simulink model "gm_uz_mpc_6ph"  (R2021a)
settings: Solver=FixedStepDiscrete  StartTime=0.0  StopTime=200*t_ADC  RelTol=1e-3
undefined symbols (not defined in the file or in its folder): IB, id_ref, iq_ref, ix_ref, iy_ref, lambda_d, lambda_q, lambda_u, lambda_x, lambda_y, Ld_over_LB, Lq_over_LB, n_rpm, omegaB, p, psi_pm_over_psiB, Rs_over_ZB, t_ADC, t_clock, Ts_times_ZB_over_Ld, Ts_times_ZB_over_Lq, Ts_times_ZB_over_Lx, Ts_times_ZB_over_Ly, v_dc, VB
libraries: nesl_utility x32, fl_lib x29, simulink x21, ee_lib x12, hdlsllib x2, spsAlphaBetaZerotodq0Lib x1
(part 2 of 4)

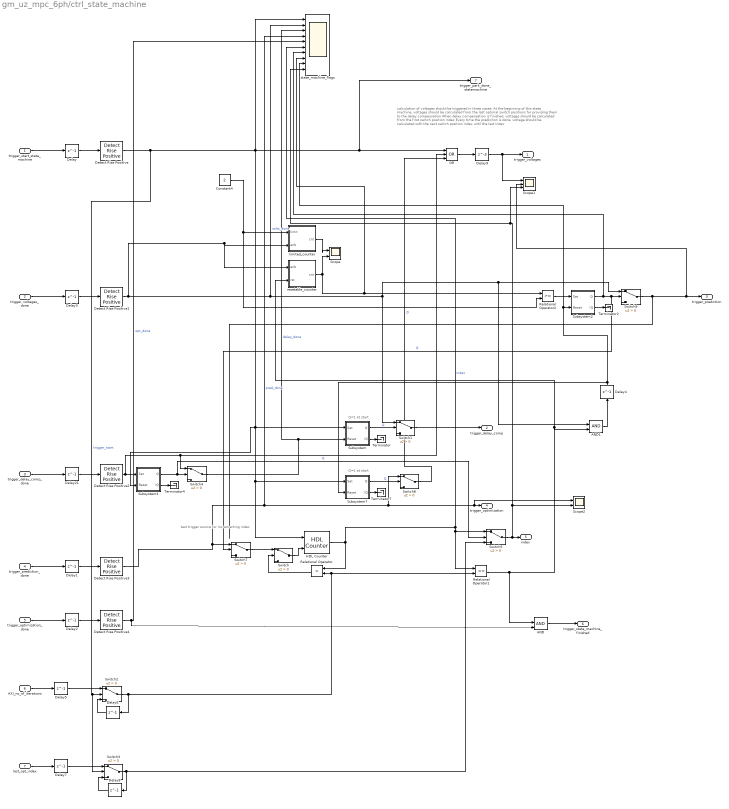
== system gm_uz_mpc_6ph/ctrl_state_machine ==
  note: Q=1 at start
  note: Q=1 at start
  note: calculation of voltages should be triggered in three cases:
      |
      | At the beginning of this state machine, voltages should be calculated from the last optimal switch positions for providing them to the delay compensation
      | When delay compensation is finished, voltages should be calculated from the first switch position index
      | Every time the prediciton is done, voltage should be calculated with the next switch position index until the last index
  note: test trigger source for incrementing index
  trigger_start_state_machine : Inport
  trigger_voltages_done : Inport  Port=2
  trigger_delay_comp_done : Inport  Port=3
  trigger_prediction_done : Inport  Port=4
  trigger_optimization_done : Inport  Port=5
  AXI_no_of_iterations : Inport  Port=6  OutDataTypeStr=uint32
  last_opt_index : Inport  Port=7  OutDataTypeStr=uint32
  AND : Logic  IconShape=distinctive  AllPortsSameDT=off  OutDataTypeStr=boolean
  AND1 : Logic  IconShape=distinctive  AllPortsSameDT=off  OutDataTypeStr=boolean
  Constant4 : Constant  Value=2  OutDataTypeStr=uint8  SampleTime=-1
  Delay{,1..8,21} (10 alike) : Delay  DelayLength=1
  Delay9 : Delay  DelayLength=3
  Detect Rise Positive{,1..4} (5 alike) : simulink/Logic and Bit Operations/Detect Rise Positive  vinit=0  OutDataTypeStr=boolean
  HDL Counter : hdlsllib/Sources/HDL Counter  CountType=Free running  CountInit=1  CountStep=1  CountMax=25  CountFromType=Initial value  CountFrom=1  CountResetPort=on  CountLoadPort=off  CountEnbPort=on  CountDirPort=off  CountHitOutputPort=off  CountDataType=Unsigned  CountWordLen=32  CountFracLen=0  CountSampTime=1
  OR : Logic  Operator=OR  Inputs=3  IconShape=distinctive  AllPortsSameDT=off  OutDataTypeStr=boolean
  Relational Operator : RelationalOperator  Operator=<  OutDataTypeStr=boolean  RndMeth=Simplest
  Relational Operator1 : RelationalOperator  Operator===  OutDataTypeStr=boolean  RndMeth=Simplest
  Relational Operator2 : RelationalOperator  OutDataTypeStr=boolean  RndMeth=Simplest
  Scope : Scope  NumInputPorts=2
  Scope1 : Scope  NumInputPorts=3
  Scope2 : Scope  NumInputPorts=2
  Subsystem : Subsystem
  Subsystem2 : Subsystem
  Subsystem4 : Subsystem
  Subsystem7 : Subsystem
  Switch{,1..5,7..9} (9 alike) : Switch  Criteria=u2 > Threshold
  Terminator{,2,4,7} (4 alike) : Terminator
  limited_counter : Subsystem
  resetable_counter : Subsystem
  state_machine_flags : Scope  NumInputPorts=10
  trigger_voltages : Outport  VectorParamsAs1DForOutWhenUnconnected=off
  trigger_delay_comp : Outport  Port=2  VectorParamsAs1DForOutWhenUnconnected=off
  trigger_prediction : Outport  Port=3  VectorParamsAs1DForOutWhenUnconnected=off
  trigger_optimization : Outport  Port=4  VectorParamsAs1DForOutWhenUnconnected=off
  index : Outport  Port=5  VectorParamsAs1DForOutWhenUnconnected=off
  trigger_state_machine_finished : Outport  Port=6  VectorParamsAs1DForOutWhenUnconnected=off
  trigger_park_done_statemachine : Outport  Port=7  VectorParamsAs1DForOutWhenUnconnected=off
  wires:
  Delay9/1 -> trigger_voltages/1, Scope1/1
  OR/1 -> Delay9/1
  Switch5/1 -> index/1, Scope2/2, state_machine_flags/10, Scope1/3
  Delay8/1 -> Switch3/3
  Delay7/1 -> Switch3/1
  Switch3/1 -> Delay8/1, Switch5/3
  last_opt_index/1 -> Delay7/1
  Delay6/1 -> Switch2/3
  Delay5/1 -> Switch2/1
  AXI_no_of_iterations/1 -> Delay5/1
  Subsystem7/1(Q) -> Switch8/2  "Q"
  Subsystem7/2(!Q) -> Terminator7/1
  Switch8/1 -> OR/3  "Q"
  Delay4/1 -> Subsystem7/2(Reset), Subsystem2/2(Reset), state_machine_flags/9
  AND1/1 -> Delay4/1
  AND/1 -> trigger_state_machine_finished/1
  Switch9/1 -> trigger_prediction/1, Scope1/2
  Relational Operator1/1 -> AND/1, resetable_counter/2(rst), AND1/2
  resetable_counter/1(cnt) -> Relational Operator2/1, state_machine_flags/8, Scope/2
  Switch7/1 -> Switch/1
  Detect Rise Positive4/1 -> AND/2, state_machine_flags/5  "opt_done"
  HDL Counter/1 -> Relational Operator/1, state_machine_flags/6, Relational Operator1/1, Switch5/1  "index"
  Switch/1 -> HDL Counter/2
  Detect Rise Positive3/1 -> trigger_optimization/1, Scope2/1, Switch8/1, state_machine_flags/4, Switch7/1  "pred_done"
  limited_counter/1(cnt) -> Scope/1
  Relational Operator2/1 -> Subsystem2/1(Set)
  Constant4/1 -> limited_counter/1(limit), Relational Operator2/2
  Subsystem2/1(Q) -> Switch9/2, Switch7/2, state_machine_flags/7  "Q"
  Subsystem2/2(!Q) -> Terminator2/1
  Delay3/1 -> Detect Rise Positive1/1
  Detect Rise Positive1/1 -> Switch1/1, Switch9/1, AND1/1, state_machine_flags/2, limited_counter/2(enb), resetable_counter/1(enb)  "volts_done"
  Switch4/1 -> Subsystem/2(Reset), state_machine_flags/3  "delay_done"
  Detect Rise Positive2/1 -> Subsystem4/1(Set), Switch4/1, OR/2
  Subsystem4/2(!Q) -> Terminator4/1
  Subsystem4/1(Q) -> Switch4/2, Switch5/2  "Q"
  trigger_prediction_done/1 -> Delay1/1
  Delay1/1 -> Detect Rise Positive3/1
  trigger_optimization_done/1 -> Delay2/1
  Delay2/1 -> Detect Rise Positive4/1
  trigger_start_state_machine/1 -> Delay/1
  Delay/1 -> Detect Rise Positive/1
  Delay21/1 -> Detect Rise Positive2/1
  trigger_delay_comp_done/1 -> Delay21/1
  trigger_voltages_done/1 -> Delay3/1
  Switch1/1 -> trigger_delay_comp/1
  Subsystem/2(!Q) -> Terminator/1
  Subsystem/1(Q) -> Switch1/2  "Q"
  Detect Rise Positive/1 -> OR/1, trigger_park_done_statemachine/1, Subsystem4/2(Reset), Subsystem/1(Set), Subsystem7/1(Set), HDL Counter/1, state_machine_flags/1, Switch2/2, Switch3/2  "trigger_start"
  Relational Operator/1 -> Switch/2
  Switch2/1 -> Relational Operator1/2, Relational Operator/2, Delay6/1

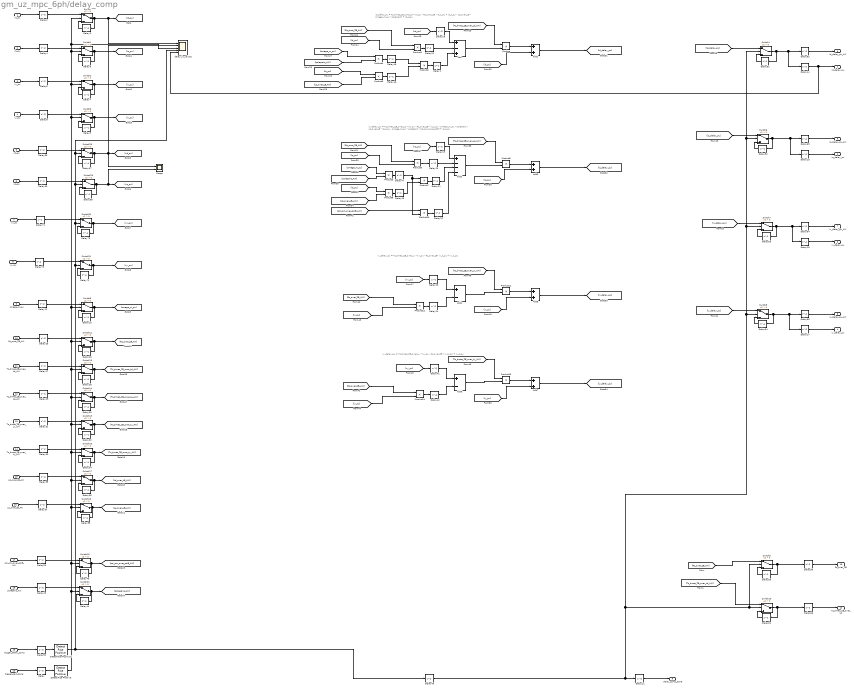
== system gm_uz_mpc_6ph/delay_comp ==
  note: id_delay_pu = Ts_times_ZB_over_Ld *(vd_pu - Rs_over_ZB * id_k_pu + iq_k_pu * Lq_over_LB * omega_m_pu * polepairs) + id_k_pu
  note: iq_delay_pu = Ts_times_ZB_over_Lq *(vq_pu - Rs_over_ZB * iq_k_pu - omega_m_pu * polepairs * Ld_over_LB * id_k_pu - omega_m_pu * polepairs * psi_pm_over_psiB) + iq_k_pu
  note: ix_delay_pu = Ts_times_ZB_over_Lx *(vx_pu - Rs_over_ZB* ix_k_pu) + ix_k_pu
  note: iy_delay_pu = Ts_times_ZB_over_Ly *(vy_pu - Rs_over_ZB * iy_k_pu) + iy_k_pu
  id_pu : Inport  OutDataTypeStr=fixdt_type_dq_currents
  iq_pu : Inport  Port=2  OutDataTypeStr=fixdt_type_dq_currents
  ix_pu : Inport  Port=3  OutDataTypeStr=fixdt_type_xy_currents
  iy_pu : Inport  Port=4  OutDataTypeStr=fixdt_type_xy_currents
  vd_pu : Inport  Port=5  OutDataTypeStr=fixdt_type_dqxy_voltages
  vq_pu : Inport  Port=6  OutDataTypeStr=fixdt_type_dqxy_voltages
  vx_pu : Inport  Port=7  OutDataTypeStr=fixdt_type_dqxy_voltages
  vy_pu : Inport  Port=8  OutDataTypeStr=fixdt_type_dqxy_voltages
  omega_m_pu : Inport  Port=9  OutDataTypeStr=fixdt_type_speed
  Rs_over_ZB_AXI : Inport  Port=10  OutDataTypeStr=fixdt_type_constants
  Ts_times_ZB_over_Ld_AXI : Inport  Port=11  OutDataTypeStr=fixdt_type_constants
  Ts_times_ZB_over_Lq_AXI : Inport  Port=12  OutDataTypeStr=fixdt_type_constants
  Ts_times_ZB_over_Lx_AXI : Inport  Port=13  OutDataTypeStr=fixdt_type_constants
  Ts_times_ZB_over_Ly_AXI : Inport  Port=14  OutDataTypeStr=fixdt_type_constants
  Ld_over_LB_AXI : Inport  Port=15  OutDataTypeStr=fixdt_type_constants
  Lq_over_LB_AXI : Inport  Port=16  OutDataTypeStr=fixdt_type_constants
  psi_pm_over_psiB_AXI : Inport  Port=17  OutDataTypeStr=fixdt_type_constants
  polepairs_AXI : Inport  Port=18  OutDataTypeStr=fixdt_type_polepairs
  trigger_delay_comp : Inport  Port=19
  trigger_park_done : Inport  Port=20
  Add : Sum  Inputs=+-+  AccumDataTypeStr=fixdt(1,27,16)
  Add{1,3,5,7} (4 alike) : Sum  AccumDataTypeStr=fixdt(1,27,24)
  Add2 : Sum  Inputs=+---  AccumDataTypeStr=fixdt(1,27,16)
  Add4 : Sum  Inputs=+-  AccumDataTypeStr=fixdt(1,27,16)
  Add6 : Sum  Inputs=+-  AccumDataTypeStr=fixdt(1,27,16)
  Delay{,2,4,6,8,10..12,14..20,23..25,27,29,31,33,35,37,39,41..43,49..50,56,59..60,62..66,71,73} (40 alike) : Delay
  Delay{1,3,5,7,9,13,21..22,26,28,30,32,34,36,38,40,44..48,51..55,57..58,61,70,72} (31 alike) : Delay  DelayLength=1
  Detect Rise Positive : simulink/Logic and Bit Operations/Detect Rise Positive  vinit=0  OutDataTypeStr=boolean
  Detect Rise Positive1 : simulink/Logic and Bit Operations/Detect Rise Positive  vinit=0  OutDataTypeStr=boolean
  Product{,1..2,4..7,9..14} (13 alike) : Product  OutDataTypeStr=fixdt(1,18,15)
  Product3 : Product  OutDataTypeStr=fixdt(1,27,16)
  Product8 : Product  OutDataTypeStr=fixdt(1,27,16)
  Scope : Scope  NumInputPorts=2
  Switch : Switch  Criteria=u2 > Threshold  OutDataTypeStr=fixdt_type_dq_currents
  Switch1 : Switch  Criteria=u2 > Threshold  OutDataTypeStr=fixdt_type_dq_currents
  Switch{4,6..10} (6 alike) : Switch  Criteria=u2 > Threshold
  Switch{12..19} (8 alike) : Switch  Criteria=u2 > Threshold  OutDataTypeStr=fixdt_type_constants
  Switch2 : Switch  Criteria=u2 > Threshold  OutDataTypeStr=fixdt_type_xy_currents
  Switch21 : Switch  Criteria=u2 > Threshold  OutDataTypeStr=fixdt_type_polepairs
  Switch{28..31} (4 alike) : Switch  Criteria=u2 > Threshold  OutDataTypeStr=fixdt_type_dqxy_voltages
  Switch3 : Switch  Criteria=u2 > Threshold  OutDataTypeStr=fixdt_type_xy_currents
  Switch5 : Switch  Criteria=u2 > Threshold  OutDataTypeStr=fixdt_type_speed
  delay_in_values : Scope  NumInputPorts=5
  id_delay_pu : Outport
  iq_delay_pu : Outport  Port=2
  ix_delay_pu : Outport  Port=3
  iy_delay_pu : Outport  Port=4
  id_delay_pu_AXI : Outport  Port=5
  iq_delay_pu_AXI : Outport  Port=6
  ix_delay_pu_AXI : Outport  Port=7
  iy_delay_pu_AXI : Outport  Port=8
  delay_comp_done : Outport  Port=9
  Rs_over_ZB : Outport  Port=10
  Ts_times_ZB_over_Ld : Outport  Port=11
  wires:
  Delay66/1 -> Ts_times_ZB_over_Ld/1
  [Ts_times_ZB_over_Ld_AXI] -> Switch10/1
  Delay61/1 -> Switch10/3
  Switch10/1 -> Delay66/1, Delay61/1
  Delay56/1 -> Rs_over_ZB/1
  Delay49/1 -> Delay11/1, Switch4/2, Switch6/2, Switch7/2, Switch8/2, Switch10/2, Switch9/2
  [Rs_over_ZB_AXI] -> Switch9/1
  Delay55/1 -> Switch9/3
  Switch9/1 -> Delay56/1, Delay55/1
  [iy_delay_pu] -> Switch8/1
  Delay54/1 -> Switch8/3
  Delay53/1 -> Switch7/3
  [ix_delay_pu] -> Switch7/1
  Delay52/1 -> Switch6/3
  Switch6/1 -> Delay63/1, Delay15/1, Delay52/1
  [iq_delay_pu] -> Switch6/1
  Delay51/1 -> Switch4/3
  [id_delay_pu] -> Switch4/1
  Detect Rise Positive1/1 -> Switch31/2, Switch30/2, Switch29/2, Switch28/2, delay_in_values/4, Delay49/1  "delay_comp done"
  Detect Rise Positive/1 -> delay_in_values/3, Switch/2, Switch1/2, Switch2/2, Switch3/2, Switch5/2, Switch12/2, Switch13/2, Switch14/2, Switch15/2, Switch16/2, Switch17/2, Switch18/2, Switch19/2, Switch21/2
  Delay50/1 -> Detect Rise Positive1/1
  trigger_delay_comp/1 -> Delay50/1
  Delay48/1 -> Product7/2
  Product8/1 -> Delay48/1
  Delay47/1 -> Product7/1, Product10/2
  Product9/1 -> Delay47/1
  Delay45/1 -> Product2/1
  Delay46/1 -> Product2/2
  Product3/1 -> Delay46/1
  Product4/1 -> Delay45/1
  Delay41/1 -> Add6/1
  Delay42/1 -> Add6/2
  Product14/1 -> Delay42/1
  [vy_pu] -> Delay41/1  "vy_pu"
  Delay24/1 -> Add4/2
  Product12/1 -> Delay24/1
  Delay23/1 -> Add4/1
  [vx_pu] -> Delay23/1  "vx_pu"
  Product6/1 -> Delay20/1
  Delay19/1 -> Add2/1
  Delay20/1 -> Add2/2
  Delay21/1 -> Add2/3
  Delay22/1 -> Add2/4
  Product10/1 -> Delay22/1
  Product7/1 -> Delay21/1
  [vq_pu] -> Delay19/1  "vq_pu"
  Delay18/1 -> Add/1
  [vd_pu] -> Delay18/1  "vd_pu"
  Delay1/1 -> Add/3
  Delay10/1 -> Add/2
  Product1/1 -> Delay10/1
  Product2/1 -> Delay1/1
  Product13/1 -> Add7/1
  [Ts_times_ZB_over_Ly_AXI] -> Product13/1  "Ts_times_ZB_over_Ly"
  [iy_pu] -> Product14/2  "iy_k_pu"
  [iy_pu] -> Add7/2  "iy_k_pu"
  Add6/1 -> Product13/2
  [Rs_over_ZB_AXI] -> Product14/1  "Rs_over_ZB"
  Product11/1 -> Add5/1
  [ix_pu] -> Add5/2  "ix_k_pu"
  Add4/1 -> Product11/2
  [Rs_over_ZB_AXI] -> Product12/1  "Rs_over_ZB"
  [ix_pu] -> Product12/2  "ix_k_pu"
  [Ts_times_ZB_over_Lx_AXI] -> Product11/1  "Ts_times_ZB_over_Lx"
  [psi_pm_over_psiB_AXI] -> Product10/1
  Product5/1 -> Add3/1
  [polepairs_AXI] -> Product9/2  "polepairs"
  [Ld_over_LB_AXI] -> Product8/2  "Ld_over_LB"
  [id_pu] -> Product8/1  "id_k_pu"
  [iq_pu] -> Add3/2  "iq_k_pu"
  [omega_m_pu] -> Product9/1  "omega_m_pu"
  Add2/1 -> Product5/2
  [Rs_over_ZB_AXI] -> Product6/1  "Rs_over_ZB"
  [iq_pu] -> Product6/2  "iq_k_pu"
  [Ts_times_ZB_over_Lq_AXI] -> Product5/1  "Ts_times_ZB_over_Lq"
  [polepairs_AXI] -> Product4/2  "polepairs"
  [omega_m_pu] -> Product4/1  "omega_m_pu"
  [Lq_over_LB_AXI] -> Product3/2  "Lq_over_LB"
  [iq_pu] -> Product3/1  "iq_k_pu"
  [id_pu] -> Product1/2  "id_k_pu"
  [Rs_over_ZB_AXI] -> Product1/1  "Rs_over_ZB"
  [id_pu] -> Add1/2  "id_k_pu"
  Product/1 -> Add1/1
  [Ts_times_ZB_over_Ld_AXI] -> Product/1  "Ts_times_ZB_over_Ld"
  Add/1 -> Product/2
  Delay17/1 -> iy_delay_pu/1
  Delay16/1 -> ix_delay_pu/1
  Delay14/1 -> id_delay_pu/1, delay_in_values/5
  Delay15/1 -> iq_delay_pu/1
  Delay62/1 -> id_delay_pu_AXI/1
  Switch7/1 -> Delay64/1, Delay16/1, Delay53/1
  Delay64/1 -> ix_delay_pu_AXI/1
  Delay65/1 -> iy_delay_pu_AXI/1
  Delay63/1 -> iq_delay_pu_AXI/1
  Switch4/1 -> Delay62/1, Delay14/1, Delay51/1
  Switch8/1 -> Delay65/1, Delay17/1, Delay54/1
  Delay11/1 -> delay_comp_done/1
  Delay30/1 -> Switch14/3
  Delay36/1 -> Switch17/3
  Delay32/1 -> Switch15/3
  Delay13/1 -> Switch5/3
  Delay40/1 -> Switch19/3
  trigger_park_done/1 -> Delay/1
  Delay39/1 -> Switch19/1
  Rs_over_ZB_AXI/1 -> Delay25/1
  Delay57/1 -> Switch28/3
  Ts_times_ZB_over_Ld_AXI/1 -> Delay27/1
  Switch1/1 -> Delay5/1, [iq_pu]
  Delay71/1 -> Switch30/1
  Ts_times_ZB_over_Lx_AXI/1 -> Delay31/1
  Switch19/1 -> Delay40/1, [psi_pm_over_psiB_AXI]
  Delay26/1 -> Switch12/3
  Switch18/1 -> [Lq_over_LB_AXI], Delay38/1
  Delay3/1 -> Switch/3
  Ts_times_ZB_over_Lq_AXI/1 -> Delay29/1
  Switch30/1 -> [vx_pu], Delay70/1
  Delay60/1 -> Switch29/1
  Delay70/1 -> Switch30/3
  vy_pu/1 -> Delay73/1
  iy_pu/1 -> Delay8/1
  iq_pu/1 -> Delay4/1
  Lq_over_LB_AXI/1 -> Delay37/1
  Switch5/1 -> Delay13/1, [omega_m_pu]
  vq_pu/1 -> Delay60/1
  Delay27/1 -> Switch13/1
  Delay6/1 -> Switch2/1
  omega_m_pu/1 -> Delay12/1
  Switch31/1 -> [vy_pu], Delay72/1
  Delay73/1 -> Switch31/1
  Delay12/1 -> Switch5/1
  Switch2/1 -> Delay7/1, [ix_pu]
  Delay4/1 -> Switch1/1
  Delay37/1 -> Switch18/1
  Delay7/1 -> Switch2/3
  Ts_times_ZB_over_Ly_AXI/1 -> Delay33/1
  Switch28/1 -> Delay57/1, [vd_pu], delay_in_values/2, Scope/1
  Delay31/1 -> Switch15/1
  Delay35/1 -> Switch17/1
  Switch/1 -> Delay3/1, [id_pu], delay_in_values/1
  Switch21/1 -> Delay44/1, [polepairs_AXI]
  id_pu/1 -> Delay2/1
  Delay58/1 -> Switch29/3
  psi_pm_over_psiB_AXI/1 -> Delay39/1
  Delay28/1 -> Switch13/3
  Switch14/1 -> Delay30/1, [Ts_times_ZB_over_Lq_AXI]
  Delay43/1 -> Switch21/1
  Delay72/1 -> Switch31/3
  polepairs_AXI/1 -> Delay43/1
  Switch3/1 -> Delay9/1, [iy_pu]
  Switch29/1 -> Delay58/1, [vq_pu], Scope/2
  Delay8/1 -> Switch3/1
  Delay29/1 -> Switch14/1
  Delay44/1 -> Switch21/3
  Delay34/1 -> Switch16/3
  Delay/1 -> Detect Rise Positive/1
  Switch13/1 -> Delay28/1, [Ts_times_ZB_over_Ld_AXI]
  Delay9/1 -> Switch3/3
  Switch17/1 -> [Ld_over_LB_AXI], Delay36/1
  Delay38/1 -> Switch18/3
  ix_pu/1 -> Delay6/1
  Switch16/1 -> [Ts_times_ZB_over_Ly_AXI], Delay34/1
  Delay2/1 -> Switch/1
  Ld_over_LB_AXI/1 -> Delay35/1
  Switch15/1 -> Delay32/1, [Ts_times_ZB_over_Lx_AXI]
  vd_pu/1 -> Delay59/1
  vx_pu/1 -> Delay71/1
  Delay33/1 -> Switch16/1
  Delay59/1 -> Switch28/1
  Delay25/1 -> Switch12/1
  Delay5/1 -> Switch1/3
  Add7/1 -> [iy_delay_pu]
  Add1/1 -> [id_delay_pu]
  Add3/1 -> [iq_delay_pu]
  Switch12/1 -> Delay26/1, [Rs_over_ZB_AXI]
  Add5/1 -> [ix_delay_pu]

== system gm_uz_mpc_6ph/inverter_machine ==
  note: 6-phase 2-level inverter
  note: electrical motor and mechanical system
  In1 : Inport
  inverter_en : Inport  Port=2
  10kHz_current : Scope
  6ph_Inverter : Subsystem
  Constant30 : Constant  Value=2*pi  SampleTime=-1
  Constant44 : Constant  Value=v_dc  SampleTime=-1
  DC_link : Subsystem
  Data Type Conversion66 : DataTypeConversion  OutDataTypeStr=double
  Demux2 : Demux  Outputs=12
  Electrical Reference1 : fl_lib/Electrical/Electrical Elements/Electrical Reference
  Gain1 : Gain  Gain=30/pi
  Gain2 : Gain  Gain=pi/30
  Gain7 : Gain  Gain=p
  Ideal Angular Velocity Source1 : fl_lib/Mechanical/Mechanical Sources/Ideal Angular Velocity Source
  Ideal Rotational Motion Sensor1 : fl_lib/Mechanical/Mechanical Sensors/Ideal Rotational Motion Sensor  wrap_angle=simscape.enum.onoff.off  offset=0 deg
  Inertia1 : fl_lib/Mechanical/Rotational Elements/Inertia  inertia=J kg*m^2  num_ports=foundation.enum.numPorts2.one  w_specify=off  w_priority=High  w=0 rad/s  w_nominal_specify=off  w_nominal_unit=rad/s  w_nominal_value=1  t_specify=off  t_priority=None  t=0 N*m  t_nominal_specify=off  t_nominal_unit=N*m  t_nominal_value=1
  Mechanical Rotational Reference1 : fl_lib/Mechanical/Rotational Elements/Mechanical Rotational Reference
  Mod : Math  Operator=mod  SaturateOnIntegerOverflow=on
  Mux8 : Mux  Inputs=6
  Open Circuit : fl_lib/Electrical/Electrical Elements/Open Circuit  v_specify=off  v_priority=None  v=0 V  v_nominal_specify=off  v_nominal_unit=V  v_nominal_value=1
      settings: SourceProductBaseCode=SS
  Open Circuit1 : fl_lib/Electrical/Electrical Elements/Open Circuit  v_specify=off  v_priority=None  v=0 V  v_nominal_specify=off  v_nominal_unit=V  v_nominal_value=1
      settings: SourceProductBaseCode=SS
  PS-Simulink Converter6 : nesl_utility/PS-Simulink Converter  PhysicalDomain=network_engine_domain  SubClassName=ps_output  LeftPortType=input  RightPortType=output  PseudoPeriodic=off  Frequencies=[]  Unit=1  AffineConversion=off
      settings: SourceProductBaseCode=PW,SS
  PS-Simulink Converter7 : nesl_utility/PS-Simulink Converter  PhysicalDomain=network_engine_domain  SubClassName=ps_output  LeftPortType=input  RightPortType=output  PseudoPeriodic=off  Frequencies=[]  Unit=1  AffineConversion=off
      settings: SourceProductBaseCode=PW,SS
  Power_Source : Subsystem
  Rate Transition : RateTransition  OutPortSampleTime=1e-6
  Rate Transition67 : RateTransition  OutPortSampleTime=0.0001
  Simscape Component : SimscapeComponentBlock  SourceFile=SixPhase_PMSM  ComponentPath=SixPhase_PMSM  ComponentVariants=SixPhase_PMSM  ComponentVariantNames=SixPhase_PMSM  ClassName=SixPhase_PMSM  SchemaVersion=1  Rs=Rs Ohm  Ld=Ld H  Lq=Lq H  Lx=Lx H  Ly=Ly H  psiPM=psi_pm Wb  np=p  theta_m_specify=off  theta_m_priority=None  theta_m=0 rad  theta_m_nominal_specify=off  theta_m_nominal_unit=rad  theta_m_nominal_value=1
      settings: CopyFcn=simscape.engine.sli.internal.componentblockcallback(gcbh,'COPY')  PreCopyFcn=simscape.engine.sli.internal.componentblockcallback(gcbh,'PRECOPY')  PreDeleteFcn=simscape.engine.sli.internal.componentblockcallback(gcbh,'PREDELETE')  InternalSimscapePortConfiguration="{\"Bottom\":[],\"Left\":[{\"id\":\"a1\",\"label\":\"a1\",\"type\":\"foundation.electrical.electrical\"},{\"id\":\"b1\",\"label\":\"b1\",\"type\":\"foundation.electrical.electrical\"},{\"id\":\"c1\",\"label\":\"c1\",\"type\":\"foundation.electrical.electrical\"},{\"id\":\"a2\",\"label\":\"a2\",\"type\":\"foundation.electrical.electrical\"},{\"id\":\"b2\",\"label\":\"b2\",\"type\":\"foundation.electrical.electrical\"},{\"id\":\"c2\",\"label\":\"c2\",\"type\":\"foundation.electrical.electrical\"},{\"id\":\"n1\",\"label\":\"n1\",\"type\":\"foundation.electrical.electrical\"},{\"id\":\"n2\",\"label\":\"n2\",\"type\":\"foundation.electrical.electrical\"}],\"Right\":[{\"id\":\"R\",\"label\":\"R\",\"type\":\"foundation.mechanical.rotational.rotational\"},{\"id\":\"C\",\"label\":\"C\",\"type\":\"foundation.mechanical.rotational.rotational\"}],\"Top\":[]}"
      mask Type: SixPhase_PMSM
  Simulink-PS Converter{,2..8,11..12,17..20} (14 alike) : nesl_utility/Simulink-PS Converter  PhysicalDomain=network_engine_domain  SubClassName=ps_input  LeftPortType=input  RightPortType=output  PseudoPeriodic=off  Frequencies=[]  NoiseDistribution=none  NoiseParameters=[]  Unit=1  AffineConversion=off  FilteringAndDerivatives=provide  SimscapeFilterOrder=1  InputFilterTimeConstant=0.001  UdotUserProvided=0
      Simulink-PS Converter settings: SourceProductBaseCode=PW,SS
      Simulink-PS Converter8 settings: SourceProductBaseCode=PW,SS
  Solver Configuration1 : nesl_utility/Solver Configuration  PhysicalDomain=network_engine_domain  SubClassName=solver  LeftPortType=input  RightPortType=generic  Tones=[]  Harmonics=[]  SimulateNoise=off  Profile=off  UseLocalSampling=off  EnableSwitchedLinearOptims=on  FrequencyDomain=off  UseCCode=off  RelTol=0.001  AbsTol=1e-06  MinStep=1e-09  ToWorkspace=off  RevertToSquareIcSolve=off  NumHomotopyIterations=100  PhasorMode=off  PhasorModeNumHarmonics=1  DoDC=off  ResidualTolerance=1e-09  UseLocalSolver=on  LocalSolverChoice=NE_BACKWARD_EULER_ADVANCER  LocalSolverSampleTime=1e-6  DoFixedCost=on  MaxNonlinIter=3  MaxModeIter=2  ComputeImpulses=off  ImpulseIterations=2  LinearAlgebra=Sparse  EquationFormulation=NE_TIME_EF  DelaysMemoryBudget=1024  AutomaticFiltering=on  FilteringTimeConstant=0.001  PartitionStorageMethod=AS_NEEDED  PartitionMemoryBudget=1024  PartitionMethod=FAST
      settings: SourceProductBaseCode=PW,SS
  n_ref : Constant  Value=n_rpm  SampleTime=-1
  i_ph : Outport
  i_dc : Outport  Port=2
  theta_el : Outport  Port=3
  omega_m : Outport  Port=4
  wires:
  inverter_en/1 -> 6ph_Inverter/1(inverter_en)
  Rate Transition67/1 -> 10kHz_current/1
  Demux2/3 -> Simulink-PS Converter5/1
  n_ref/1 -> Gain2/1
  6ph_Inverter/6(i_6) -> Mux8/6  "i_c2"
  Rate Transition/1 -> Data Type Conversion66/1
  Demux2/8 -> Simulink-PS Converter19/1
  6ph_Inverter/4(i_4) -> Mux8/4  "i_a2"
  Demux2/10 -> Simulink-PS Converter3/1
  Demux2/2 -> Simulink-PS Converter4/1
  Demux2/1 -> Simulink-PS Converter2/1
  Constant44/1 -> Simulink-PS Converter/1
  6ph_Inverter/1(i_1) -> Mux8/1  "i_a1"
  Demux2/7 -> Simulink-PS Converter18/1
  Constant30/1 -> Mod/2
  Demux2/9 -> Simulink-PS Converter20/1
  Demux2/4 -> Simulink-PS Converter6/1
  Demux2/12 -> Simulink-PS Converter12/1
  In1/1 -> Rate Transition/1
  DC_link/1(u_dc_link_measured) -> [u_dc_link]
  6ph_Inverter/2(i_2) -> Mux8/2  "i_b1"
  Mod/1 -> [theta_el], theta_el/1
  Data Type Conversion66/1 -> Demux2/1
  PS-Simulink Converter7/1 -> Gain7/1  "theta_m"
  6ph_Inverter/13(i_dc) -> [i_dc], i_dc/1
  Demux2/5 -> Simulink-PS Converter7/1
  Demux2/6 -> Simulink-PS Converter17/1
  Gain1/1 -> [n_RPM]
  PS-Simulink Converter6/1 -> Gain1/1  "omega_m"
  6ph_Inverter/5(i_5) -> Mux8/5  "i_b2"
  6ph_Inverter/3(i_3) -> Mux8/3  "i_c1"
  Gain7/1 -> Mod/1  "theta_el"
  Gain2/1 -> Simulink-PS Converter8/1, omega_m/1, [omega_m]
  Demux2/11 -> Simulink-PS Converter11/1
  Mux8/1 -> [i_ph], i_ph/1, Rate Transition67/1
  connections:
  Simulink-PS Converter20/RConn1 -- 6ph_Inverter/LConn9
  Simulink-PS Converter2/RConn1 -- 6ph_Inverter/LConn1
  Simulink-PS Converter18/RConn1 -- 6ph_Inverter/LConn7
  6ph_Inverter/RConn1 -- Simscape Component/LConn1
  6ph_Inverter/LConn13 -- DC_link/RConn1
  Power_Source/RConn1 -- DC_link/LConn1
  Simulink-PS Converter8/RConn1 -- Ideal Angular Velocity Source1/RConn1
  Simulink-PS Converter4/RConn1 -- 6ph_Inverter/LConn2
  6ph_Inverter/RConn5 -- Simscape Component/LConn5
  Simulink-PS Converter5/RConn1 -- 6ph_Inverter/LConn3
  PS-Simulink Converter7/LConn1 -- Ideal Rotational Motion Sensor1/RConn3
  Simulink-PS Converter19/RConn1 -- 6ph_Inverter/LConn8
  Simulink-PS Converter/RConn1 -- Power_Source/LConn1
  6ph_Inverter/RConn2 -- Simscape Component/LConn2
  Simscape Component/LConn8 -- Open Circuit1/LConn1
  Simulink-PS Converter7/RConn1 -- 6ph_Inverter/LConn5
  Simscape Component/LConn7 -- Open Circuit/LConn1
  Simulink-PS Converter17/RConn1 -- 6ph_Inverter/LConn6
  6ph_Inverter/RConn4 -- Simscape Component/LConn4
  Simulink-PS Converter12/RConn1 -- 6ph_Inverter/LConn12
  6ph_Inverter/LConn14 -- DC_link/RConn2
  Simscape Component/LConn3 -- 6ph_Inverter/RConn3
  Simulink-PS Converter11/RConn1 -- 6ph_Inverter/LConn11
  Simulink-PS Converter3/RConn1 -- 6ph_Inverter/LConn10
  Simscape Component/RConn2 -- Ideal Angular Velocity Source1/RConn2 -- Ideal Rotational Motion Sensor1/RConn1 -- Mechanical Rotational Reference1/LConn1
  Inertia1/LConn1 -- Ideal Angular Velocity Source1/LConn1 -- Simscape Component/RConn1 -- Ideal Rotational Motion Sensor1/LConn1
  Simscape Component/LConn6 -- 6ph_Inverter/RConn6
  Solver Configuration1/RConn1 -- Power_Source/RConn2 -- DC_link/LConn2 -- Electrical Reference1/LConn1
  PS-Simulink Converter6/LConn1 -- Ideal Rotational Motion Sensor1/RConn2
  Simulink-PS Converter6/RConn1 -- 6ph_Inverter/LConn4

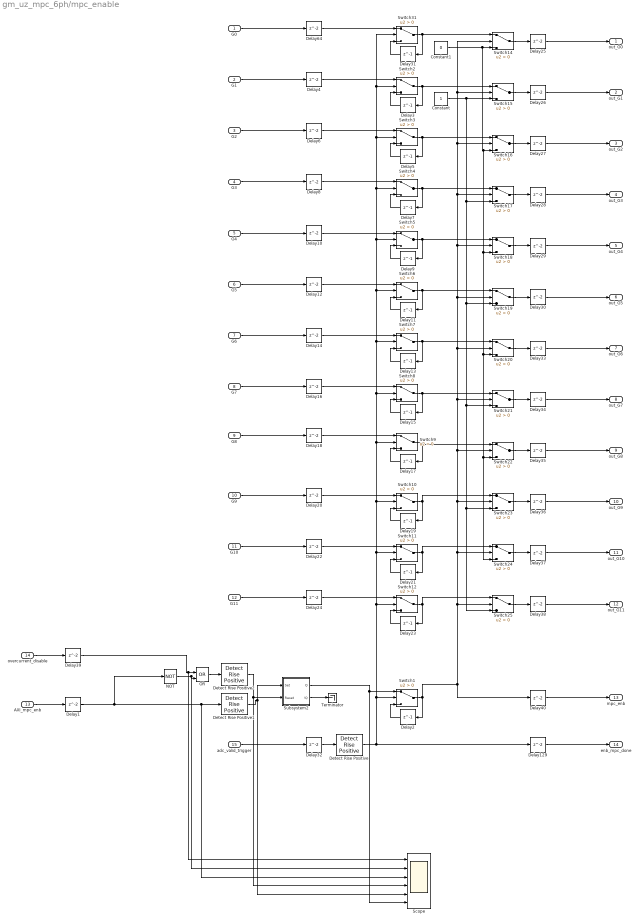
== system gm_uz_mpc_6ph/mpc_enable ==
  G0 : Inport
  G1 : Inport  Port=2
  G2 : Inport  Port=3
  G3 : Inport  Port=4
  G4 : Inport  Port=5
  G5 : Inport  Port=6
  G6 : Inport  Port=7
  G7 : Inport  Port=8
  G8 : Inport  Port=9
  G9 : Inport  Port=10
  G10 : Inport  Port=11
  G11 : Inport  Port=12
  AXI_mpc_enb : Inport  Port=13
  overcurrent_disable : Inport  Port=14
  adc_valid_trigger : Inport  Port=15  OutDataTypeStr=boolean
  Constant : Constant  OutDataTypeStr=boolean  SampleTime=-1
  Constant1 : Constant  Value=0  OutDataTypeStr=boolean  SampleTime=-1
  Delay{1,4,6,8,10,12,14,16,18,20,22,24..30,32..40,64,129} (29 alike) : Delay
  Delay{2..3,5,7,9,11,13,15,17,19,21,23,31} (13 alike) : Delay  DelayLength=1
  Detect Rise Positive : simulink/Logic and Bit Operations/Detect Rise Positive  vinit=0  OutDataTypeStr=boolean
  Detect Rise Positive1 : simulink/Logic and Bit Operations/Detect Rise Positive  vinit=0  OutDataTypeStr=boolean
  Detect Rise Positive2 : simulink/Logic and Bit Operations/Detect Rise Positive  vinit=0  OutDataTypeStr=boolean
  NOT : Logic  Operator=NOT  IconShape=distinctive  AllPortsSameDT=off  OutDataTypeStr=boolean
  OR : Logic  Operator=OR  IconShape=distinctive  AllPortsSameDT=off  OutDataTypeStr=boolean
  Scope : Scope  NumInputPorts=6
  Subsystem2 : Subsystem
  Switch{1..12,14..25,31} (25 alike) : Switch  Criteria=u2 > Threshold
  Terminator : Terminator
  out_G0 : Outport
  out_G1 : Outport  Port=2
  out_G2 : Outport  Port=3
  out_G3 : Outport  Port=4
  out_G4 : Outport  Port=5
  out_G5 : Outport  Port=6
  out_G6 : Outport  Port=7
  out_G7 : Outport  Port=8
  out_G8 : Outport  Port=9
  out_G9 : Outport  Port=10
  out_G10 : Outport  Port=11
  out_G11 : Outport  Port=12
  mpc_enb : Outport  Port=13  OutDataTypeStr=boolean  LockScale=on
  enb_mpc_done : Outport  Port=14  OutDataTypeStr=boolean  LockScale=on
  wires:
  Subsystem2/2(!Q) -> Terminator/1
  Delay40/1 -> mpc_enb/1
  Delay1/1 -> NOT/1, Detect Rise Positive1/1, Scope/3
  Delay39/1 -> OR/1, Scope/1
  overcurrent_disable/1 -> Delay39/1
  NOT/1 -> OR/2, Scope/2
  OR/1 -> Detect Rise Positive2/1
  Detect Rise Positive2/1 -> Scope/4, Subsystem2/2(Reset)
  Detect Rise Positive1/1 -> Scope/5, Subsystem2/1(Set)
  Subsystem2/1(Q) -> Switch1/1, Scope/6
  Constant/1 -> Switch15/3, Switch17/3, Switch19/3, Switch21/3, Switch23/3, Switch25/3
  Switch21/1 -> Delay34/1
  Delay37/1 -> out_G10/1
  Delay34/1 -> out_G7/1
  Switch24/1 -> Delay37/1
  Switch25/1 -> Delay38/1
  Delay38/1 -> out_G11/1
  Delay36/1 -> out_G9/1
  Delay33/1 -> out_G6/1
  Switch23/1 -> Delay36/1
  Delay35/1 -> out_G8/1
  Switch20/1 -> Delay33/1
  Switch22/1 -> Delay35/1
  Delay30/1 -> out_G5/1
  Switch18/1 -> Delay29/1
  Switch19/1 -> Delay30/1
  Delay29/1 -> out_G4/1
  Delay27/1 -> out_G2/1
  Switch17/1 -> Delay28/1
  Delay28/1 -> out_G3/1
  Switch16/1 -> Delay27/1
  Switch1/1 -> Delay2/1, Switch14/2, Switch15/2, Switch16/2, Switch17/2, Switch18/2, Switch19/2, Switch20/2, Switch21/2, Switch22/2, Switch23/2, Switch24/2, Switch25/2, Delay40/1
  Delay26/1 -> out_G1/1
  Switch15/1 -> Delay26/1
  Constant1/1 -> Switch14/3, Switch16/3, Switch18/3, Switch20/3, Switch22/3, Switch24/3
  Delay25/1 -> out_G0/1
  Switch14/1 -> Delay25/1
  G11/1 -> Delay24/1
  Delay24/1 -> Switch12/1
  Switch12/1 -> Delay23/1, Switch25/1
  Delay23/1 -> Switch12/3
  G10/1 -> Delay22/1
  Delay22/1 -> Switch11/1
  Switch11/1 -> Delay21/1, Switch24/1
  Delay21/1 -> Switch11/3
  G9/1 -> Delay20/1
  Delay20/1 -> Switch10/1
  Switch10/1 -> Switch23/1, Delay19/1
  Delay19/1 -> Switch10/3
  G8/1 -> Delay18/1
  Delay18/1 -> Switch9/1
  Switch9/1 -> Delay17/1, Switch22/1
  Delay17/1 -> Switch9/3
  G7/1 -> Delay16/1
  Delay16/1 -> Switch8/1
  Switch8/1 -> Delay15/1, Switch21/1
  Delay15/1 -> Switch8/3
  G6/1 -> Delay14/1
  Delay14/1 -> Switch7/1
  Switch7/1 -> Delay13/1, Switch20/1
  Delay13/1 -> Switch7/3
  G5/1 -> Delay12/1
  Delay12/1 -> Switch6/1
  Switch6/1 -> Delay11/1, Switch19/1
  Delay11/1 -> Switch6/3
  G4/1 -> Delay10/1
  Delay10/1 -> Switch5/1
  Switch5/1 -> Delay9/1, Switch18/1
  Delay9/1 -> Switch5/3
  G3/1 -> Delay8/1
  Delay8/1 -> Switch4/1
  Switch4/1 -> Delay7/1, Switch17/1
  Delay7/1 -> Switch4/3
  G2/1 -> Delay6/1
  Delay6/1 -> Switch3/1
  Switch3/1 -> Delay5/1, Switch16/1
  Delay5/1 -> Switch3/3
  Detect Rise Positive/1 -> Switch1/2, Switch12/2, Switch11/2, Switch10/2, Switch9/2, Switch8/2, Switch7/2, Switch6/2, Switch5/2, Switch4/2, Switch3/2, Switch2/2, Switch31/2, Delay129/1
  G1/1 -> Delay4/1
  Delay4/1 -> Switch2/1
  Switch2/1 -> Delay3/1, Switch15/1
  Delay3/1 -> Switch2/3
  Delay2/1 -> Switch1/3
  AXI_mpc_enb/1 -> Delay1/1
  Delay31/1 -> Switch31/3
  Switch31/1 -> Delay31/1, Switch14/1
  Delay32/1 -> Detect Rise Positive/1
  Delay64/1 -> Switch31/1
  Delay129/1 -> enb_mpc_done/1
  G0/1 -> Delay64/1
  adc_valid_trigger/1 -> Delay32/1

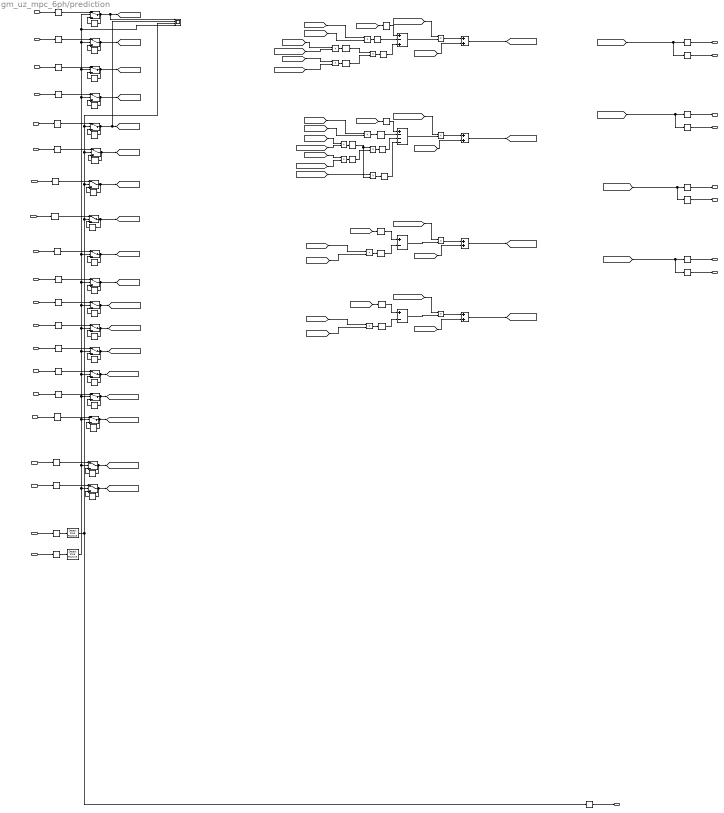
== system gm_uz_mpc_6ph/prediction ==
  note: id_delay_pu = Ts_times_ZB_over_Ld *(vd_pu - Rs_over_ZB * id_k_pu + iq_k_pu * Lq_over_LB * omega_m_pu * polepairs) + id_k_pu
  note: iq_delay_pu = Ts_times_ZB_over_Lq *(vq_pu - Rs_over_ZB * iq_k_pu - omega_m_pu * polepairs * Ld_over_LB * id_k_pu - omega_m_pu * polepairs * psi_pm_over_psiB) + iq_k_pu
  note: ix_delay_pu = Ts_times_ZB_over_Lx *(vx_pu - Rs_over_ZB* ix_k_pu) + ix_k_pu
  note: iy_delay_pu = Ts_times_ZB_over_Ly *(vy_pu - Rs_over_ZB * iy_k_pu) + iy_k_pu
  note: voltages are triggered every iteration
  id_delay_pu : Inport  OutDataTypeStr=fixdt_type_dq_currents
  iq_delay_pu : Inport  Port=2  OutDataTypeStr=fixdt_type_dq_currents
  ix_delay_pu : Inport  Port=3  OutDataTypeStr=fixdt_type_dq_currents
  iy_delay_pu : Inport  Port=4  OutDataTypeStr=fixdt_type_dq_currents
  vd_pu : Inport  Port=5  OutDataTypeStr=fixdt_type_dqxy_voltages
  vq_pu : Inport  Port=6  OutDataTypeStr=fixdt_type_dqxy_voltages
  vx_pu : Inport  Port=7  OutDataTypeStr=fixdt_type_dqxy_voltages
  vy_pu : Inport  Port=8  OutDataTypeStr=fixdt_type_dqxy_voltages
  omega_m_pu : Inport  Port=9  OutDataTypeStr=fixdt_type_speed
  Rs_over_ZB_AXI : Inport  Port=10  OutDataTypeStr=fixdt_type_constants
  Ts_times_ZB_over_Ld_AXI : Inport  Port=11  OutDataTypeStr=fixdt_type_constants
  Ts_times_ZB_over_Lq_AXI : Inport  Port=12  OutDataTypeStr=fixdt_type_constants
  Ts_times_ZB_over_Lx_AXI : Inport  Port=13  OutDataTypeStr=fixdt_type_constants
  Ts_times_ZB_over_Ly_AXI : Inport  Port=14  OutDataTypeStr=fixdt_type_constants
  Ld_over_LB_AXI : Inport  Port=15  OutDataTypeStr=fixdt_type_constants
  Lq_over_LB_AXI : Inport  Port=16  OutDataTypeStr=fixdt_type_constants
  psi_pm_over_psiB_AXI : Inport  Port=17  OutDataTypeStr=fixdt_type_constants
  polepairs_AXI : Inport  Port=18  OutDataTypeStr=fixdt_type_polepairs
  trigger_prediction : Inport  Port=19
  trigger_delay_comp_done : Inport  Port=20
  Add : Sum  Inputs=+-+  AccumDataTypeStr=fixdt(1,27,16)
  Add{1,3,5,7} (4 alike) : Sum  AccumDataTypeStr=fixdt(1,27,24)
  Add2 : Sum  Inputs=+---  AccumDataTypeStr=fixdt(1,27,16)
  Add4 : Sum  Inputs=+-  AccumDataTypeStr=fixdt(1,27,16)
  Add6 : Sum  Inputs=+-  AccumDataTypeStr=fixdt(1,27,16)
  Delay{,2,4,6,8,11..12,14..17,25,27,29,31,33,35,37,39,43,50,59..60,62..65,71,73} (29 alike) : Delay
  Delay{1,3,5,7,9..10,13,18..24,26,28,30,32,34,36,38,40..42,44..48,57..58,70,72} (33 alike) : Delay  DelayLength=1
  Detect Rise Positive : simulink/Logic and Bit Operations/Detect Rise Positive  vinit=0  OutDataTypeStr=boolean
  Detect Rise Positive1 : simulink/Logic and Bit Operations/Detect Rise Positive  vinit=0  OutDataTypeStr=boolean
  Product{,1..2,4..7,9..14} (13 alike) : Product  OutDataTypeStr=fixdt(1,18,15)
  Product3 : Product  OutDataTypeStr=fixdt(1,27,16)
  Product8 : Product  OutDataTypeStr=fixdt(1,27,16)
  Scope : Scope  NumInputPorts=4
  Switch{,1..3} (4 alike) : Switch  Criteria=u2 > Threshold  OutDataTypeStr=fixdt_type_dq_currents
  Switch{12..19} (8 alike) : Switch  Criteria=u2 > Threshold  OutDataTypeStr=fixdt_type_constants
  Switch21 : Switch  Criteria=u2 > Threshold  OutDataTypeStr=fixdt_type_polepairs
  Switch{28..31} (4 alike) : Switch  Criteria=u2 > Threshold  OutDataTypeStr=fixdt_type_dqxy_voltages
  Switch5 : Switch  Criteria=u2 > Threshold  OutDataTypeStr=fixdt_type_speed
  id_pred_pu : Outport
  iq_pred_pu : Outport  Port=2
  ix_pred_pu : Outport  Port=3
  iy_pred_pu : Outport  Port=4
  id_pred_pu_AXI : Outport  Port=5
  iq_pred_pu_AXI : Outport  Port=6
  ix_pred_pu_AXI : Outport  Port=7
  iy_pred_pu_AXI : Outport  Port=8
  prediction_done : Outport  Port=9
  wires:
  Detect Rise Positive/1 -> Switch/2, Scope/4, Switch1/2, Switch2/2, Switch3/2, Switch5/2, Switch12/2, Switch13/2, Switch14/2, Switch15/2, Switch16/2, Switch17/2, Switch18/2, Switch19/2, Switch21/2
  Delay50/1 -> Detect Rise Positive1/1
  trigger_prediction/1 -> Delay50/1
  Detect Rise Positive1/1 -> Switch28/2, Scope/3, Switch29/2, Switch30/2, Switch31/2, Delay11/1  "delay_comp done"
  Delay48/1 -> Product7/2
  Product8/1 -> Delay48/1
  Delay47/1 -> Product7/1, Product10/2
  Product9/1 -> Delay47/1
  Delay45/1 -> Product2/1
  Delay46/1 -> Product2/2
  Product3/1 -> Delay46/1
  Product4/1 -> Delay45/1
  Delay41/1 -> Add6/1
  Delay42/1 -> Add6/2
  Product14/1 -> Delay42/1
  [vy_pu] -> Delay41/1  "vy_pu"
  Delay24/1 -> Add4/2
  Product12/1 -> Delay24/1
  Delay23/1 -> Add4/1
  [vx_pu] -> Delay23/1  "vx_pu"
  Product6/1 -> Delay20/1
  Delay19/1 -> Add2/1
  Delay20/1 -> Add2/2
  Delay21/1 -> Add2/3
  Delay22/1 -> Add2/4
  Product10/1 -> Delay22/1
  Product7/1 -> Delay21/1
  [vq_pu] -> Delay19/1  "vq_pu"
  Delay18/1 -> Add/1
  [vd_pu] -> Delay18/1  "vd_pu"
  Delay1/1 -> Add/3
  Delay10/1 -> Add/2
  Product1/1 -> Delay10/1
  Product2/1 -> Delay1/1
  Product13/1 -> Add7/1
  [Ts_times_ZB_over_Ly_AXI] -> Product13/1  "Ts_times_ZB_over_Ly"
  [iy_pu] -> Product14/2  "iy_k_pu"
  [iy_pu] -> Add7/2  "iy_k_pu"
  Add6/1 -> Product13/2
  [Rs_over_ZB_AXI] -> Product14/1  "Rs_over_ZB"
  Product11/1 -> Add5/1
  [ix_pu] -> Add5/2  "ix_k_pu"
  Add4/1 -> Product11/2
  [Rs_over_ZB_AXI] -> Product12/1  "Rs_over_ZB"
  [ix_pu] -> Product12/2  "ix_k_pu"
  [Ts_times_ZB_over_Lx_AXI] -> Product11/1  "Ts_times_ZB_over_Lx"
  [psi_pm_over_psiB_AXI] -> Product10/1
  Product5/1 -> Add3/1
  [polepairs_AXI] -> Product9/2  "polepairs"
  [Ld_over_LB_AXI] -> Product8/2  "Ld_over_LB"
  [id_pu] -> Product8/1  "id_k_pu"
  [iq_pu] -> Add3/2  "iq_k_pu"
  [omega_m_pu] -> Product9/1  "omega_m_pu"
  Add2/1 -> Product5/2
  [Rs_over_ZB_AXI] -> Product6/1  "Rs_over_ZB"
  [iq_pu] -> Product6/2  "iq_k_pu"
  [Ts_times_ZB_over_Lq_AXI] -> Product5/1  "Ts_times_ZB_over_Lq"
  [polepairs_AXI] -> Product4/2  "polepairs"
  [omega_m_pu] -> Product4/1  "omega_m_pu"
  [Lq_over_LB_AXI] -> Product3/2  "Lq_over_LB"
  [iq_pu] -> Product3/1  "iq_k_pu"
  [id_pu] -> Product1/2  "id_k_pu"
  [Rs_over_ZB_AXI] -> Product1/1  "Rs_over_ZB"
  [id_pu] -> Add1/2  "id_k_pu"
  Product/1 -> Add1/1
  [Ts_times_ZB_over_Ld_AXI] -> Product/1  "Ts_times_ZB_over_Ld"
  Add/1 -> Product/2
  Delay17/1 -> iy_pred_pu/1
  Delay16/1 -> ix_pred_pu/1
  Delay14/1 -> id_pred_pu/1
  Delay15/1 -> iq_pred_pu/1
  Delay62/1 -> id_pred_pu_AXI/1
  [ix_delay_pu] -> Delay64/1, Delay16/1
  Delay64/1 -> ix_pred_pu_AXI/1
  Delay65/1 -> iy_pred_pu_AXI/1
  Delay63/1 -> iq_pred_pu_AXI/1
  [id_delay_pu] -> Delay62/1, Delay14/1
  [iq_delay_pu] -> Delay63/1, Delay15/1
  [iy_delay_pu] -> Delay65/1, Delay17/1
  Delay11/1 -> prediction_done/1
  Delay30/1 -> Switch14/3
  Delay36/1 -> Switch17/3
  Delay32/1 -> Switch15/3
  Delay13/1 -> Switch5/3
  Delay40/1 -> Switch19/3
  trigger_delay_comp_done/1 -> Delay/1
  Delay39/1 -> Switch19/1
  Rs_over_ZB_AXI/1 -> Delay25/1
  Delay57/1 -> Switch28/3
  Ts_times_ZB_over_Ld_AXI/1 -> Delay27/1
  Switch1/1 -> Delay5/1, [iq_pu]
  Delay71/1 -> Switch30/1
  Ts_times_ZB_over_Lx_AXI/1 -> Delay31/1
  Switch19/1 -> Delay40/1, [psi_pm_over_psiB_AXI]
  Delay26/1 -> Switch12/3
  Switch18/1 -> [Lq_over_LB_AXI], Delay38/1
  Delay3/1 -> Switch/3
  Ts_times_ZB_over_Lq_AXI/1 -> Delay29/1
  Switch30/1 -> [vx_pu], Delay70/1
  Delay60/1 -> Switch29/1
  Delay70/1 -> Switch30/3
  vy_pu/1 -> Delay73/1
  iy_delay_pu/1 -> Delay8/1
  iq_delay_pu/1 -> Delay4/1
  Lq_over_LB_AXI/1 -> Delay37/1
  Switch5/1 -> Delay13/1, [omega_m_pu]
  vq_pu/1 -> Delay60/1
  Delay27/1 -> Switch13/1
  Delay6/1 -> Switch2/1
  omega_m_pu/1 -> Delay12/1
  Switch31/1 -> [vy_pu], Delay72/1
  Delay73/1 -> Switch31/1
  Delay12/1 -> Switch5/1
  Switch2/1 -> Delay7/1, [ix_pu]
  Delay4/1 -> Switch1/1
  Delay37/1 -> Switch18/1
  Delay7/1 -> Switch2/3
  Ts_times_ZB_over_Ly_AXI/1 -> Delay33/1
  Switch28/1 -> Delay57/1, [vd_pu], Scope/2
  Delay31/1 -> Switch15/1
  Delay35/1 -> Switch17/1
  Switch/1 -> Delay3/1, [id_pu], Scope/1
  Switch21/1 -> Delay44/1, [polepairs_AXI]
  id_delay_pu/1 -> Delay2/1
  Delay58/1 -> Switch29/3
  psi_pm_over_psiB_AXI/1 -> Delay39/1
  Delay28/1 -> Switch13/3
  Switch14/1 -> Delay30/1, [Ts_times_ZB_over_Lq_AXI]
  Delay43/1 -> Switch21/1
  Delay72/1 -> Switch31/3
  polepairs_AXI/1 -> Delay43/1
  Switch3/1 -> Delay9/1, [iy_pu]
  Switch29/1 -> Delay58/1, [vq_pu]
  Delay8/1 -> Switch3/1
  Delay29/1 -> Switch14/1
  Delay44/1 -> Switch21/3
  Delay34/1 -> Switch16/3
  Delay/1 -> Detect Rise Positive/1
  Switch13/1 -> Delay28/1, [Ts_times_ZB_over_Ld_AXI]
  Delay9/1 -> Switch3/3
  Switch17/1 -> [Ld_over_LB_AXI], Delay36/1
  Delay38/1 -> Switch18/3
  ix_delay_pu/1 -> Delay6/1
  Switch16/1 -> [Ts_times_ZB_over_Ly_AXI], Delay34/1
  Delay2/1 -> Switch/1
  Ld_over_LB_AXI/1 -> Delay35/1
  Switch15/1 -> Delay32/1, [Ts_times_ZB_over_Lx_AXI]
  vd_pu/1 -> Delay59/1
  vx_pu/1 -> Delay71/1
  Delay33/1 -> Switch16/1
  Delay59/1 -> Switch28/1
  Delay25/1 -> Switch12/1
  Delay5/1 -> Switch1/3
  Add7/1 -> [iy_delay_pu]
  Add1/1 -> [id_delay_pu]
  Add3/1 -> [iq_delay_pu]
  Switch12/1 -> Delay26/1, [Rs_over_ZB_AXI]
  Add5/1 -> [ix_delay_pu]

== system gm_uz_mpc_6ph/pu_omega_m ==
  in1 : Inport  OutDataTypeStr=fixdt(1,24,11)
  AXI_pu_conv_in : Inport  Port=2  OutDataTypeStr=fixdt(0,18,18)
  adc_valid_trigger : Inport  Port=3  OutDataTypeStr=boolean
  Delay{32,64,127..129} (5 alike) : Delay
  Delay31 : Delay  DelayLength=1
  Detect Rise Positive : simulink/Logic and Bit Operations/Detect Rise Positive  vinit=0  OutDataTypeStr=boolean
  Product23 : Product  OutDataTypeStr=fixdt(1,24,11)
  Switch31 : Switch  Criteria=u2 > Threshold
  out1 : Outport
  pu_conv_done : Outport  Port=2  OutDataTypeStr=boolean  LockScale=on
  out1_AXI : Outport  Port=3
  wires:
  Delay127/1 -> out1/1
  Product23/1 -> Delay128/1, Delay127/1
  Detect Rise Positive/1 -> Switch31/2, Delay129/1
  Delay31/1 -> Switch31/3
  Switch31/1 -> Delay31/1, Product23/2
  Delay32/1 -> Detect Rise Positive/1
  Delay128/1 -> out1_AXI/1
  Delay64/1 -> Switch31/1
  AXI_pu_conv_in/1 -> Product23/1
  Delay129/1 -> pu_conv_done/1
  in1/1 -> Delay64/1
  adc_valid_trigger/1 -> Delay32/1

== system gm_uz_mpc_6ph/pu_omega_m1 ==
  in1 : Inport  OutDataTypeStr=fixdt(1,24,11)
  AXI_pu_conv_in : Inport  Port=2  OutDataTypeStr=fixdt(0,18,18)
  adc_valid_trigger : Inport  Port=3  OutDataTypeStr=boolean
  Delay{32,64,127..129} (5 alike) : Delay
  Delay31 : Delay  DelayLength=1
  Detect Rise Positive : simulink/Logic and Bit Operations/Detect Rise Positive  vinit=0  OutDataTypeStr=boolean
  Product23 : Product  OutDataTypeStr=fixdt(1,24,11)
  Switch31 : Switch  Criteria=u2 > Threshold
  out1 : Outport
  pu_conv_done : Outport  Port=2  OutDataTypeStr=boolean  LockScale=on
  out1_AXI : Outport  Port=3
  wires:
  Delay127/1 -> out1/1
  Product23/1 -> Delay128/1, Delay127/1
  Detect Rise Positive/1 -> Switch31/2, Delay129/1
  Delay31/1 -> Switch31/3
  Switch31/1 -> Delay31/1, Product23/2
  Delay32/1 -> Detect Rise Positive/1
  Delay128/1 -> out1_AXI/1
  Delay64/1 -> Switch31/1
  AXI_pu_conv_in/1 -> Product23/1
  Delay129/1 -> pu_conv_done/1
  in1/1 -> Delay64/1
  adc_valid_trigger/1 -> Delay32/1

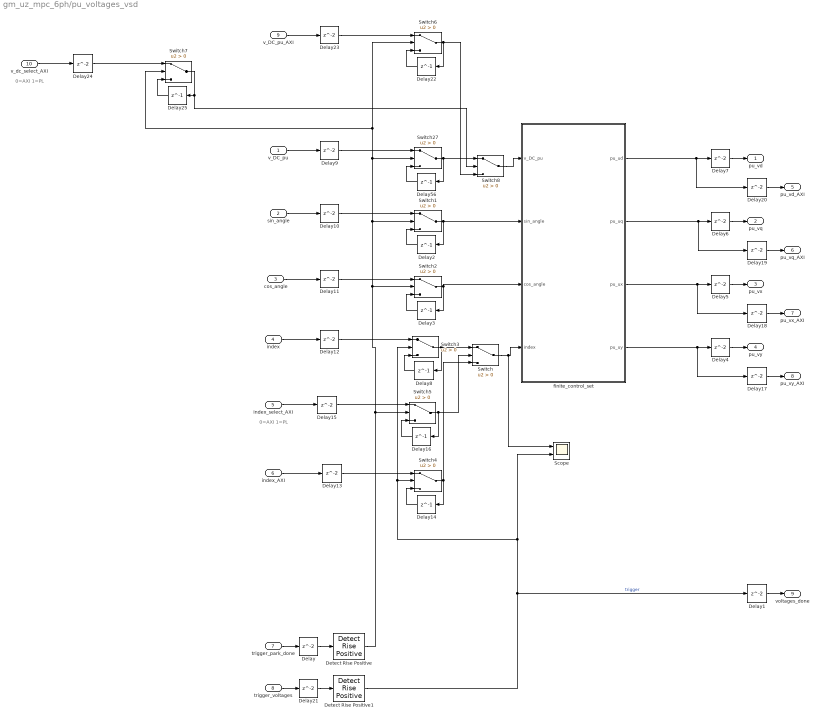
== system gm_uz_mpc_6ph/pu_voltages_vsd ==
  note: 0=AXI 1=PL
  note: 0=AXI 1=PL
  v_DC_pu : Inport  OutDataTypeStr=fixdt_type_constants
  sin_angle : Inport  Port=2  OutDataTypeStr=fixdt_type_sin_cos
  cos_angle : Inport  Port=3  OutDataTypeStr=fixdt_type_sin_cos
  index : Inport  Port=4
  index_select_AXI : Inport  Port=5
  index_AXI : Inport  Port=6
  trigger_park_done : Inport  Port=7
  trigger_voltages : Inport  Port=8
  v_DC_pu_AXI : Inport  Port=9  OutDataTypeStr=fixdt_type_constants
  v_dc_select_AXI : Inport  Port=10
  Delay{,1,4..7,9..11,17..21,23} (15 alike) : Delay
  Delay{12..13,15,24} (4 alike) : Delay  InitialCondition=1
  Delay{8,14,16,25} (4 alike) : Delay  DelayLength=1  InitialCondition=1
  Delay{2..3,22,56} (4 alike) : Delay  DelayLength=1
  Detect Rise Positive : simulink/Logic and Bit Operations/Detect Rise Positive  vinit=0  OutDataTypeStr=boolean
  Detect Rise Positive1 : simulink/Logic and Bit Operations/Detect Rise Positive  vinit=0  OutDataTypeStr=boolean
  Scope : Scope  NumInputPorts=2
  Switch : Switch  Criteria=u2 > Threshold
  Switch1 : Switch  Criteria=u2 > Threshold  OutDataTypeStr=fixdt_type_sin_cos
  Switch2 : Switch  Criteria=u2 > Threshold  OutDataTypeStr=fixdt_type_sin_cos
  Switch27 : Switch  Criteria=u2 > Threshold  OutDataTypeStr=fixdt_type_constants
  Switch{3..5,7} (4 alike) : Switch  Criteria=u2 > Threshold  OutDataTypeStr=fixdt_type_polepairs
  Switch6 : Switch  Criteria=u2 > Threshold  OutDataTypeStr=fixdt_type_constants
  Switch8 : Switch  Criteria=u2 > Threshold
  finite_control_set : MATLAB Function  TreatAsAtomicUnit=on
  pu_vd : Outport
  pu_vq : Outport  Port=2
  pu_vx : Outport  Port=3
  pu_vy : Outport  Port=4
  pu_vd_AXI : Outport  Port=5
  pu_vq_AXI : Outport  Port=6
  pu_vx_AXI : Outport  Port=7
  pu_vy_AXI : Outport  Port=8
  voltages_done : Outport  Port=9
  wires:
  Switch8/1 -> finite_control_set/1(v_DC_pu)
  Detect Rise Positive/1 -> Switch1/2, Switch27/2, Switch6/2, Switch7/2, Switch2/2, Switch5/2
  Delay24/1 -> Switch7/1
  Switch7/1 -> Delay25/1, Switch8/2
  Delay25/1 -> Switch7/3
  v_dc_select_AXI/1 -> Delay24/1
  Delay23/1 -> Switch6/1
  v_DC_pu_AXI/1 -> Delay23/1
  Delay22/1 -> Switch6/3
  Switch6/1 -> Delay22/1, Switch8/3
  Switch/1 -> finite_control_set/4(index), Scope/1
  Delay21/1 -> Detect Rise Positive1/1
  trigger_voltages/1 -> Delay21/1
  Delay1/1 -> voltages_done/1
  Detect Rise Positive1/1 -> Delay1/1, Switch4/2, Switch3/2, Scope/2  "trigger"
  Delay18/1 -> pu_vx_AXI/1
  Delay20/1 -> pu_vd_AXI/1
  Delay19/1 -> pu_vq_AXI/1
  Delay17/1 -> pu_vy_AXI/1
  Delay15/1 -> Switch5/1
  Switch5/1 -> Delay16/1, Switch/2
  index_select_AXI/1 -> Delay15/1
  Delay16/1 -> Switch5/3
  Delay13/1 -> Switch4/1
  Switch4/1 -> Delay14/1, Switch/3
  index_AXI/1 -> Delay13/1
  Delay14/1 -> Switch4/3
  Delay12/1 -> Switch3/1
  Delay11/1 -> Switch2/1
  Delay10/1 -> Switch1/1
  Delay9/1 -> Switch27/1
  Delay8/1 -> Switch3/3
  index/1 -> Delay12/1
  Switch3/1 -> Switch/1, Delay8/1
  Delay7/1 -> pu_vd/1
  Delay6/1 -> pu_vq/1
  Delay5/1 -> pu_vx/1
  Delay4/1 -> pu_vy/1
  Switch2/1 -> Delay3/1, finite_control_set/3(cos_angle)
  Delay3/1 -> Switch2/3
  cos_angle/1 -> Delay11/1
  Switch1/1 -> Delay2/1, finite_control_set/2(sin_angle)
  Delay2/1 -> Switch1/3
  sin_angle/1 -> Delay10/1
  Switch27/1 -> Switch8/1, Delay56/1
  v_DC_pu/1 -> Delay9/1
  Delay56/1 -> Switch27/3
  Delay/1 -> Detect Rise Positive/1
  trigger_park_done/1 -> Delay/1
  finite_control_set/4(pu_uy) -> Delay4/1, Delay17/1
  finite_control_set/3(pu_ux) -> Delay5/1, Delay18/1
  finite_control_set/2(pu_uq) -> Delay6/1, Delay19/1
  finite_control_set/1(pu_ud) -> Delay7/1, Delay20/1

== system gm_uz_mpc_6ph/uz_current_limit ==
  ia1_SI : Inport  OutDataTypeStr=fixdt(1, 27, 15)  PortDimensions=1  SampleTime=1e-08
  ib1_SI : Inport  Port=2  OutDataTypeStr=fixdt(1, 27, 15)  PortDimensions=1  SampleTime=1e-08
  ic1_SI : Inport  Port=3  OutDataTypeStr=fixdt(1, 27, 15)  PortDimensions=1  SampleTime=1e-08
  ia2_SI : Inport  Port=4  OutDataTypeStr=fixdt(1, 27, 15)  PortDimensions=1  SampleTime=1e-08
  ib2_SI : Inport  Port=5  OutDataTypeStr=fixdt(1, 27, 15)  PortDimensions=1  SampleTime=1e-08
  ic2_SI : Inport  Port=6  OutDataTypeStr=fixdt(1, 27, 15)  PortDimensions=1  SampleTime=1e-08
  i_max_ampere_AXI : Inport  Port=7  OutDataTypeStr=fixdt(1, 27, 15)  PortDimensions=1  SampleTime=1e-08
  trigger : Inport  Port=8  OutDataTypeStr=boolean  PortDimensions=1  SampleTime=1e-08
  Abs{,1..5} (6 alike) : Abs  SampleTime=1e-08  OutDataTypeStr=fixdt(1, 27, 15)
  Delay{,1..16,31} (18 alike) : Delay  DelayLength=double(1)  InitialCondition=0  SampleTime=1e-08
  Detect Rise Positive : simulink/Logic and Bit Operations/Detect Rise Positive  vinit=0  OutDataTypeStr=boolean
  OR : Logic  Operator=OR  Inputs=6  AllPortsSameDT=off  OutDataTypeStr=boolean  SampleTime=1e-08
  Relational Operator{,1..5} (6 alike) : RelationalOperator  Operator=>  OutDataTypeStr=boolean  SampleTime=1e-08  RndMeth=Nearest
  Switch{1..6,31} (7 alike) : Switch  Criteria=u2 > Threshold  Threshold=double(0)  OutDataTypeStr=fixdt(1, 27, 15)  SampleTime=1e-08
  current_limit_violated : Outport  SampleTime=1e-08  VectorParamsAs1DForOutWhenUnconnected=off
  current_limit_violated_AXI : Outport  Port=2  SampleTime=1e-08  VectorParamsAs1DForOutWhenUnconnected=off
  done : Outport  Port=3  SampleTime=1e-08  VectorParamsAs1DForOutWhenUnconnected=off
  wires:
  ia1_SI/1 -> Delay7/1
  ib1_SI/1 -> Delay6/1
  ic1_SI/1 -> Delay5/1
  ia2_SI/1 -> Delay4/1
  ib2_SI/1 -> Delay3/1
  ic2_SI/1 -> Delay2/1
  i_max_ampere_AXI/1 -> Delay1/1
  trigger/1 -> Delay/1
  Abs/1 -> Relational Operator/1
  Abs1/1 -> Relational Operator1/1
  Abs2/1 -> Relational Operator2/1
  Abs3/1 -> Relational Operator3/1
  Abs4/1 -> Relational Operator4/1
  Abs5/1 -> Relational Operator5/1
  Delay/1 -> Detect Rise Positive/1
  Delay1/1 -> Switch31/1
  Delay10/1 -> Switch3/3
  Delay11/1 -> Switch6/3
  Delay12/1 -> Switch4/3
  Delay13/1 -> Switch5/3
  Delay14/1 -> current_limit_violated/1
  Delay15/1 -> current_limit_violated_AXI/1
  Delay16/1 -> done/1
  Delay2/1 -> Switch6/1
  Delay3/1 -> Switch5/1
  Delay31/1 -> Switch31/3
  Delay4/1 -> Switch4/1
  Delay5/1 -> Switch3/1
  Delay6/1 -> Switch2/1
  Delay7/1 -> Switch1/1
  Delay8/1 -> Switch1/3
  Delay9/1 -> Switch2/3
  Detect Rise Positive/1 -> Switch6/2, Switch5/2, Switch4/2, Switch31/2, Switch3/2, Switch2/2, Switch1/2, Delay16/1
  OR/1 -> Delay15/1, Delay14/1
  Relational Operator/1 -> OR/1
  Relational Operator1/1 -> OR/2
  Relational Operator2/1 -> OR/3
  Relational Operator3/1 -> OR/4
  Relational Operator4/1 -> OR/5
  Relational Operator5/1 -> OR/6
  Switch1/1 -> Abs/1, Delay8/1
  Switch2/1 -> Abs1/1, Delay9/1
  Switch3/1 -> Abs2/1, Delay10/1
  Switch31/1 -> Relational Operator5/2, Relational Operator4/2, Relational Operator3/2, Relational Operator2/2, Relational Operator1/2, Relational Operator/2, Delay31/1
  Switch4/1 -> Abs3/1, Delay12/1
  Switch5/1 -> Abs4/1, Delay13/1
  Switch6/1 -> Abs5/1, Delay11/1
